simulink model "MPCHalo"  (R2019b)
settings: Solver=ode45  StartTime=0.0  StopTime=simTime  RelTol=1e-4
values from neighbouring files (symbols this model uses):
  a = zeros(2,1)    [initHaloMRMPC.m]
  b = zeros(2,1)    [initHaloMRMPC.m]
  c = zeros(2,1)    [initHaloMRMPC.m]
  delta = 0.1    [initHaloMRMPC.m]
  disturbance = 1    [initHaloMRMPC.m]
  Gsc = 1360.8    [initHaloMRMPC.m]
  k = 0.1    [initHaloMRMPC.m]
  L2 = 1.1556    [initHaloMRMPC.m]
  mu = 0.012149    [initHaloMRMPC.m]
  Omega = 1.8636    [initHaloMRMPC.m]
  Omega_z = Omega    (= 1.8636)    [initHaloMRMPC.m]
  phi = 0    [initHaloMRMPC.m]
  ref_select = 1    [initHaloMRMPC.m]
  Rotate_w = 0.1    [initHaloMRMPC.m]
  satValue = inf    [initHaloMRMPC.m]
  sped = 300000    [initHaloMRMPC.m]
  srp = 1    [initHaloMRMPC.m]
  Ts = delta    (= 0.1)    [initHaloMRMPC.m]
  u0 = [0;0;0]    [initHaloMRMPC.m]
  x0 = Seq + [ho1;diffho1]    [initHaloMRMPC.m]
  zeta = 0.9252    [initHaloMRMPC.m]
libraries: vrlib x3, mpclib x1, simulink x1
settings Model: Creator=mohd-  LastModifiedBy=mohd-

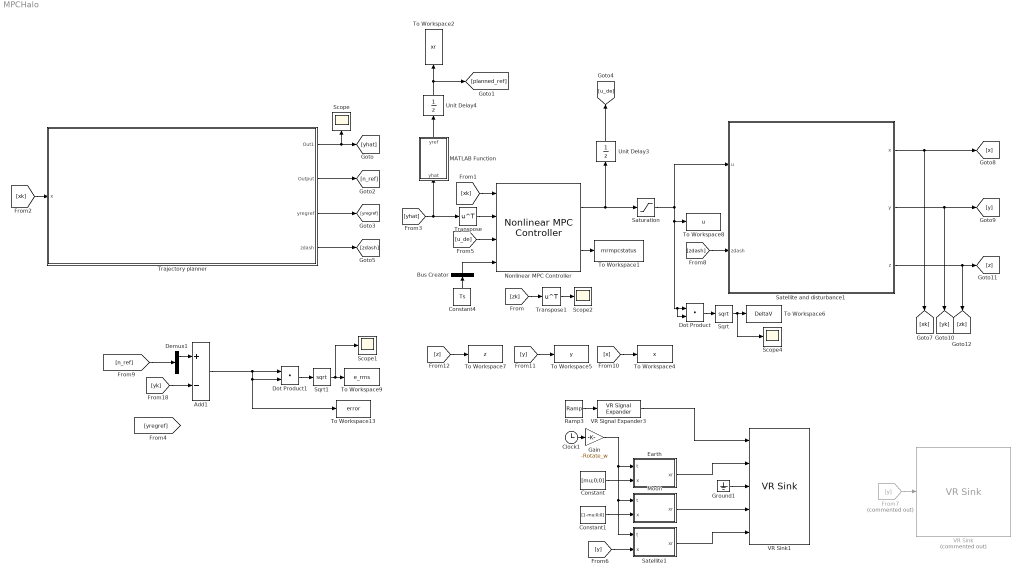
== system MPCHalo ==
  Add1 : Sum  Inputs=+-
  Bus Creator : BusCreator  Inputs=1  OutDataTypeStr=Bus: myBusObject  NonVirtualBus=on
      settings: InheritFromInputs=off
  Clock1 : Clock
  Constant : Constant  Value=[mu;0;0]
  Constant1 : Constant  Value=[1-mu;0;0]
  Constant4 : Constant  Value=Ts
  Demux1 : Demux  Outputs=[3 3]
  Dot Product : DotProduct  InputSameDT=on  OutDataTypeStr=Inherit: Inherit via internal rule
  Dot Product1 : DotProduct  InputSameDT=on  OutDataTypeStr=Inherit: Inherit via internal rule
  Earth : MATLAB Function  TreatAsAtomicUnit=on
  From7 : From  Commented=on  GotoTag=y
  Gain : Gain  Gain=-Rotate_w
  Ground1 : Ground
  MATLAB Function : MATLAB Function  TreatAsAtomicUnit=on
  Moon : MATLAB Function  TreatAsAtomicUnit=on
  Nonlinear MPC Controller : mpclib/Nonlinear MPC Controller  SCDEnableBlockLinearizationSpecification=on  nlmpcobj=nlobj  UseObjectTs=off  TsControl=delta  md_enabled=off  mvtarget_enabled=off  param_enabled=on  cost_enabled=off  mvseq_enabled=off  stateseq_enabled=off  ovseq_enabled=off  slack_enabled=off  status_enabled=on  ov_min=off  ov_max=off  mv_min=off  mv_max=off  mvrate_min=off  mvrate_max=off  state_min=off  state_max=off  ov_weight=off  mv_weight=off  mvrate_weight=off  ecr_weight=off  nlp_initialize=off
      settings: SourceProductName=Model Predictive Control Toolbox
  Ramp3 : simulink/Sources/Ramp  slope=0.4632  start=0  InitialOutput=0
  Satellite and disturbance1 : Subsystem
  Satellite1 : MATLAB Function  TreatAsAtomicUnit=on
  Saturation : Saturate  UpperLimit=satValue  LowerLimit=-satValue
  Scope{,1..2,4} (4 alike) : Scope
  Sqrt : Sqrt  SaturateOnIntegerOverflow=on
  Sqrt1 : Sqrt  SaturateOnIntegerOverflow=on
  To Workspace1 : ToWorkspace  VariableName=mrmpcstatus  SampleTime=10^-3
  To Workspace13 : ToWorkspace  VariableName=error  SampleTime=10^-3
  To Workspace2 : ToWorkspace  VariableName=xr  SampleTime=delta
  To Workspace4 : ToWorkspace  VariableName=x  SampleTime=10^-3
  To Workspace5 : ToWorkspace  VariableName=y  SampleTime=10^-3
  To Workspace6 : ToWorkspace  VariableName=DeltaV  SampleTime=10^-3
  To Workspace7 : ToWorkspace  VariableName=z  SampleTime=10^-3
  To Workspace8 : ToWorkspace  VariableName=u  SampleTime=10^-3
  To Workspace9 : ToWorkspace  VariableName=e_rms  SampleTime=delta
  Trajectory planner : Subsystem
  Transpose : Math  Operator=transpose  SignedPower=off  SaturateOnIntegerOverflow=on
  Transpose1 : Math  Operator=transpose  SignedPower=off  SaturateOnIntegerOverflow=on
  Unit Delay3 : UnitDelay  InitialCondition=u0  SampleTime=delta  HasFrameUpgradeWarning=on
  Unit Delay4 : UnitDelay  InitialCondition=x0  SampleTime=delta  HasFrameUpgradeWarning=on
  VR Signal Expander3 : vrlib/VR Signal Expander  outwidth=4  outidx=[4]
      settings: SourceProductName=Simulink
  VR Sink : vrlib/VR Sink  Commented=on  InstantiateOnLoad=on  SampleTime=-1  ViewEnable=on  RemoteChange=off  RemoteView=off  FieldsWritten=Satellite.translation.3.1.1.double  WorldFileName=satellite.wrl  WorldDescription=HaloMRMPC  AutoView=on  VideoDimensions=[]  AllowVariableSize=off  FigureProperties="{'Position', 'Name', 'Viewpoint', 'CameraBound', 'CameraDirection', 'CameraPosition', 'CameraUpVector', 'ZoomFactor', 'Antialiasing', 'Headlight', 'Lighting', 'NavPanel', 'Sound', 'StatusBar', 'Stereo3D', 'Stereo3DCameraOffset', 'Stereo3DHIT', 'ToolBar', 'Textures', 'Transparency', 'Triad', 'Wireframe', 'NavZones', 'NavMode', 'NavSpeed', 'CaptureFileFormat', 'CaptureFileName', 'Record2DCompressMethod', 'Record2DCompressQuality', 'Record2D', 'Record2DFileName', 'Record2DFPS'; [5.0000000000000000e+00   9.2000000000000000e+01   5.7600000000000000e+02   3.5000000000000000e+02], 'HaloMRMPC', 'View on Moon', 'on', [0.0000000000000000e+00   0.0000000000000000e+00  -1.0000000000000000e+00], [0.0000000000000000e+00   0.0000000000000000e+00   0.0000000000000000e+00], [0.0000000000000000e+00   1.0000000000000000e+00   0.0000000000000000e+00], [1.0000000000000000e+00], 'on', 'on', 'on', 'halfbar', 'on', 'on', 'off', [1.0000000149011612e-01], [0.0000000000000000e+00], 'on', 'on', 'on', 'none', 'off', 'off', 'fly', 'normal', 'tif', '%f_anim_%n.tif', 'auto', [7.5000000000000000e+01], 'off', '%f_anim_%n.avi', 'auto'}"
      settings: SourceProductName=Simulink
  VR Sink1 : vrlib/VR Sink  InstantiateOnLoad=on  SampleTime=-1  ViewEnable=on  RemoteChange=off  RemoteView=off  FieldsWritten=Earth.rotation.4.1.1.double#Earth.translation.3.1.1.double#Moon.rotation.4.1.1.double#Moon.translation.3.1.1.double#Satellite.translation.3.1.1.double  WorldFileName=satellite.wrl  WorldDescription=HaloMRMPC  AutoView=off  VideoDimensions=[]  AllowVariableSize=off
      settings: SourceProductName=Simulink
  wires:
  [z] -> To Workspace7/1
  [x] -> To Workspace4/1
  [y] -> To Workspace5/1
  Satellite and disturbance1/3(z) -> [z], [zk]
  Satellite and disturbance1/2(y) -> [yk], [y]
  Satellite and disturbance1/1(x) -> [xk], [x]
  Unit Delay3/1 -> [u_de]
  [u_de] -> Nonlinear MPC Controller/3
  [xk] -> Nonlinear MPC Controller/1
  Constant4/1 -> Bus Creator/1
  Bus Creator/1 -> Nonlinear MPC Controller/4
  Transpose/1 -> Nonlinear MPC Controller/2
  [zk] -> Transpose1/1
  Transpose1/1 -> Scope2/1
  [yk] -> Add1/2
  Dot Product/1 -> Sqrt/1
  Sqrt1/1 -> Scope1/1, To Workspace9/1
  Trajectory planner/1(Out1) -> [yhat], Scope/1
  [xk] -> Trajectory planner/1(x)
  MATLAB Function/1(yref) -> Unit Delay4/1
  Unit Delay4/1 -> [planned_ref], To Workspace2/1
  [yhat] -> MATLAB Function/1(yhat), Transpose/1
  Nonlinear MPC Controller/1 -> Unit Delay3/1, Saturation/1
  Saturation/1 -> Dot Product/1, Dot Product/2, To Workspace8/1, Satellite and disturbance1/1(u)
  Nonlinear MPC Controller/2 -> To Workspace1/1
  Sqrt/1 -> To Workspace6/1, Scope4/1
  Trajectory planner/2(Output) -> [n_ref]
  Dot Product1/1 -> Sqrt1/1
  Constant/1 -> Earth/2(x)
  Gain/1 -> Earth/1(t), Satellite1/1(t), Moon/1(t)
  Constant1/1 -> Moon/2(x)
  Clock1/1 -> Gain/1
  [y] -> Satellite1/2(x)
  Ramp3/1 -> VR Signal Expander3/1
  Satellite1/1(xr) -> VR Sink1/5
  Moon/1(xr) -> VR Sink1/4
  Earth/1(xr) -> VR Sink1/2
  VR Signal Expander3/1 -> VR Sink1/1
  Ground1/1 -> VR Sink1/3
  From7/1 -> VR Sink/1
  Trajectory planner/3("yregref ") -> [yregref]
  Trajectory planner/4("zdash ") -> [zdash]
  [zdash] -> Satellite and disturbance1/2("zdash ")
  [n_ref] -> Demux1/1
  Demux1/1 -> Add1/1
  Add1/1 -> To Workspace13/1, Dot Product1/2, Dot Product1/1

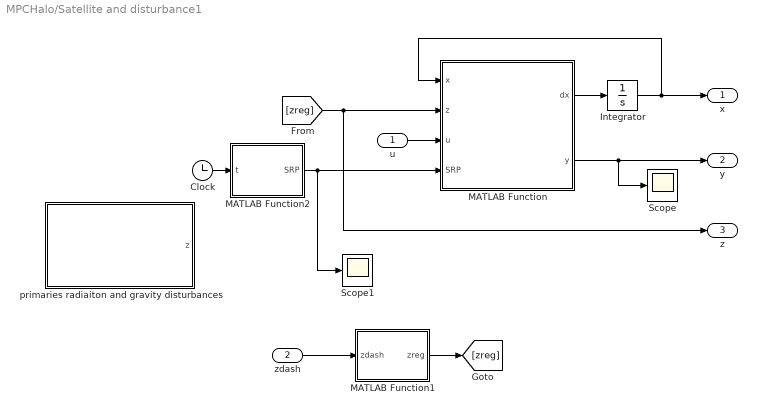
== system MPCHalo/Satellite and disturbance1 ==
  u : Inport
  "zdash " : Inport  Port=2
  Clock : Clock
  Integrator : Integrator  InitialCondition=x0
  MATLAB Function : MATLAB Function  TreatAsAtomicUnit=on
  MATLAB Function1 : MATLAB Function  TreatAsAtomicUnit=on
  MATLAB Function2 : MATLAB Function  TreatAsAtomicUnit=on
  Scope : Scope
  Scope1 : Scope
  primaries radiaiton and gravity disturbances : Subsystem
  x : Outport
  y : Outport  Port=2
  z : Outport  Port=3
  wires:
  Integrator/1 -> x/1, MATLAB Function/1(x)
  MATLAB Function/1(dx) -> Integrator/1
  MATLAB Function/2(y) -> Scope/1, y/1
  u/1 -> MATLAB Function/3(u)
  MATLAB Function1/1(zreg) -> [zreg]
  "zdash "/1 -> MATLAB Function1/1(zdash)
  [zreg] -> z/1, MATLAB Function/2(z)
  MATLAB Function2/1(SRP) -> Scope1/1, MATLAB Function/4(SRP)
  Clock/1 -> MATLAB Function2/1(t)

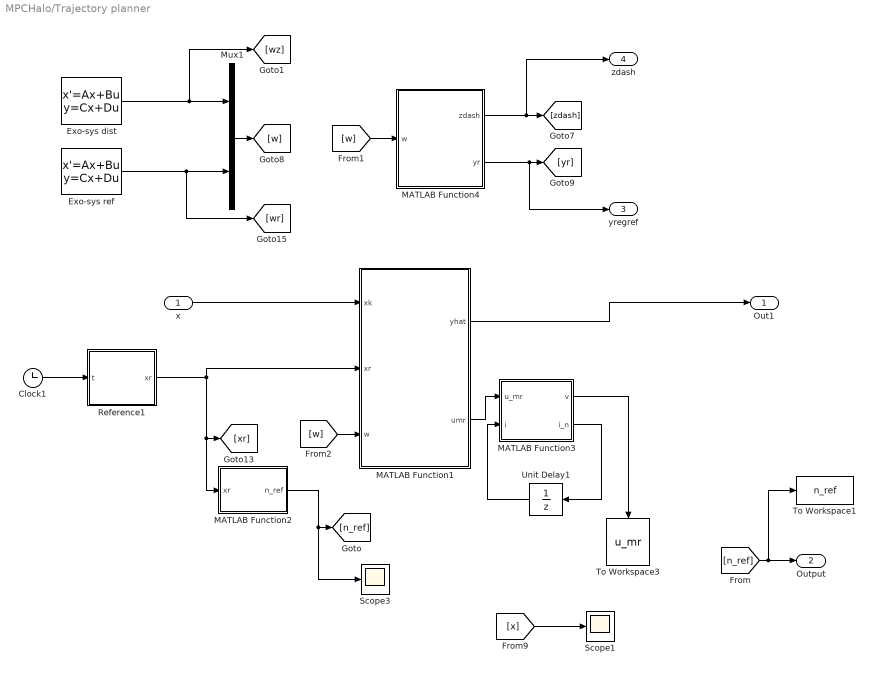
== system MPCHalo/Trajectory planner ==
  x : Inport
  Clock1 : Clock
  Exo-sys dist : StateSpace  A=[0 -1;1 0]  B=[0;0]  C=eye(2)  D=zeros(2,1)  InitialCondition=[1;0]
  "Exo-sys ref " : StateSpace  A=[0 -Omega;Omega 0]  B=[0;0]  C=eye(2)  D=zeros(2,1)  InitialCondition=[1;0]
  MATLAB Function1 : MATLAB Function  TreatAsAtomicUnit=on  SystemSampleTime=2*delta
  MATLAB Function2 : MATLAB Function  TreatAsAtomicUnit=on
  MATLAB Function3 : MATLAB Function  TreatAsAtomicUnit=on  SystemSampleTime=delta
  MATLAB Function4 : MATLAB Function  TreatAsAtomicUnit=on
  Mux1 : Mux  Inputs=2
  Reference1 : MATLAB Function  TreatAsAtomicUnit=on
  Scope1 : Scope
  Scope3 : Scope
  To Workspace1 : ToWorkspace  VariableName=n_ref  SampleTime=10^-3
  To Workspace3 : ToWorkspace  VariableName=u_mr  SampleTime=10^-3
  Unit Delay1 : UnitDelay  InitialCondition=1  SampleTime=delta  HasFrameUpgradeWarning=on
  Out1 : Outport
  Output : Outport  Port=2
  "yregref " : Outport  Port=3
  "zdash " : Outport  Port=4
  wires:
  MATLAB Function1/1(yhat) -> Out1/1
  Clock1/1 -> Reference1/1(t)
  x/1 -> MATLAB Function1/1(xk)
  MATLAB Function2/1(n_ref) -> Scope3/1, [n_ref]
  Unit Delay1/1 -> MATLAB Function3/2(i)
  MATLAB Function1/2(umr) -> MATLAB Function3/1(u_mr)
  [x] -> Scope1/1
  Reference1/1(xr) -> MATLAB Function2/1(xr), [xr], MATLAB Function1/2(xr)
  MATLAB Function3/2(i_n) -> Unit Delay1/1
  MATLAB Function3/1(v) -> To Workspace3/1
  [n_ref] -> To Workspace1/1, Output/1
  MATLAB Function4/1(zdash) -> "zdash "/1, [zdash]
  MATLAB Function4/2(yr) -> "yregref "/1, [yr]
  Mux1/1 -> [w]
  Exo-sys dist/1 -> [wz], Mux1/1
  [w] -> MATLAB Function4/1(w)
  "Exo-sys ref "/1 -> [wr], Mux1/2
  [w] -> MATLAB Function1/3(w)

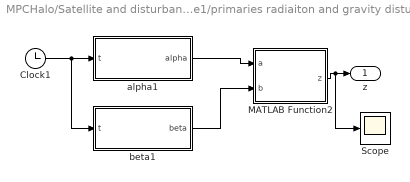
== system MPCHalo/Satellite and disturbance1/primaries radiaiton and gravity disturbances ==
  Clock1 : Clock
  MATLAB Function2 : MATLAB Function  TreatAsAtomicUnit=on
  Scope : Scope
  alpha1 : MATLAB Function  TreatAsAtomicUnit=on
  beta1 : MATLAB Function  TreatAsAtomicUnit=on
  z : Outport
  wires:
  Clock1/1 -> beta1/1(t), alpha1/1(t)
  beta1/1(beta) -> MATLAB Function2/2(b)
  alpha1/1(alpha) -> MATLAB Function2/1(a)
  MATLAB Function2/1(z) -> Scope/1, z/1

== matlab function MPCHalo/Trajectory planner/MATLAB Function2 ==
  data: xr input; n_ref output
function n_ref = fcn(xr)

n_ref = xr(:,1);

== matlab function MPCHalo/MATLAB Function ==
  data: yhat input; yref output
function yref = fcn(yhat)

yref = yhat(:,1);

== matlab function MPCHalo/Earth ==
  data: t input; xr output; x input
function xr = Rotate(t,x)
%#codegen

th = t;

R = [cos(th) sin(th) 0;
     -sin(th) cos(th) 0;
     0 0 1];
xr = R*x;

== matlab function MPCHalo/Trajectory planner/MATLAB Function1 ==
  data: yhat output; xk input; umr output; xr input; mu parameter; delta parameter; c parameter; w input; k parameter; e parameter; a parameter; b parameter; Omega parameter; disturbance parameter; L2 parameter
function [yhat, umr] = mrcontrol(xk,xr, mu,delta,c, w,k, e, a, b, Omega, disturbance, L2)

Tz = [b(1)*e 0;0 0;0 -b(1)*e;mu*(1-mu)*a(1)*e 0];
Tr = [k*(1-c(1)+Omega^2)/(2*Omega) 0;0 -k;-k 0];
S2 = [0 -Omega;Omega 0];
Seq = [L2;0;0];
if disturbance == 1
    wz = w(1:2);
else
    wz = zeros(2,1);
end
wr = w(3:4);
pi = [-Tr*wr + Seq;-Tr*S2*wr];

% ref1 = xr(:,1);
% ref2 = xr(:,2);
ref1 = pi;
ref2 = ref1;

u = zeros(3,2);
yhat = zeros(6,4); % 3 outputs for 4 small time intervals (2*delta)
x_t = xk;

delta_b = delta;
%% First step 

Ad = [ 1, 0, 0, delta_b, 0, 0; ...
      0, 1, 0, 0, delta_b,  0; ...
      0, 0, 1, 0, 0, delta_b; ...
      0, 0, 0, 1, 0,  0; ...
      0, 0, 0, 0, 1, 0; ...
      0, 0, 0, 0, 0, 1];
Am = Ad^2;
  
Bd = [delta_b^2/2 0 0;0 delta_b^2/2 0;0 0 delta_b^2/2; ...
       delta_b 0 0;0 delta_b 0; 0 0 delta_b];

Bm = [Ad*Bd Bd]; 
Cm = [eye(3) zeros(3)];

u1 = pinv(Bm)*(ref1-Am*xk);  
u11 = u1(1); 
u21 = u1(2);
u31 = u1(3);
u12 = u1(4);
u22 = u1(5);
u32 = u1(6);

u_1 = [u11 u12;u21 u22;u31 u32];

%% Second step 
xk1 = Am*xk + Bm*u1;  
u2 = pinv(Bm)*(ref2-Am*xk1); 

u11 = u2(1); 
u21 = u2(2);
u31 = u2(3);
u12 = u2(4);
u22 = u2(5);
u32 = u2(6);

u_2 = [u11 u12;u21 u22;u31 u32];

%% States planning step

x_1 = pi(1);
x_2 = pi(2);
x_3 = pi(3);
xd_1 = pi(4);
xd_2 = pi(5);


f2 = [x_1 + 2*xd_2 - (mu*(mu + x_1 - 1))/((mu + x_1 - 1)^2 + x_2^2 + x_3^2)^(3/2) + ((mu + x_1)*(mu - 1))/((mu + x_1)^2 + x_2^2 + x_3^2)^(3/2);
    x_2 - 2*xd_1 - (mu*x_2)/((mu + x_1 - 1)^2 + x_2^2 + x_3^2)^(3/2) + (x_2*(mu - 1))/((mu + x_1)^2 + x_2^2 + x_3^2)^(3/2);
    (x_3*(mu - 1))/((mu + x_1)^2 + x_2^2 + x_3^2)^(3/2) - (mu*x_3)/((mu + x_1 - 1)^2 + x_2^2 + x_3^2)^(3/2)];

P44 = -2*((x_1+mu)^2+x_2^2+x_3^2)/((x_1+mu)^2+x_2^2+x_3^2)^(5/2) - 2*((x_1-1+mu)^2+x_2^2+x_3^2)/((x_1-1+mu)^2+x_2^2+x_3^2)^(5/2);
P54 = 3*(x_2*(x_1+mu))/((x_1+mu)^2+x_2^2+x_3^2)^(5/2) - 3*(x_2*(x_1-1+mu))/((x_1-1+mu)^2+x_2^2+x_3^2)^(5/2);
P64 = 3*(x_3*(x_1+mu))/((x_1+mu)^2+x_2^2+x_3^2)^(5/2) - 3*x_3*((x_1-1+mu))/((x_1-1+mu)^2+x_2^2+x_3^2)^(5/2);

P2 = [ 2*x_1 + 2*xd_2, x_1,  x_2, P44;
    2*x_2 - 2*xd_1, x_2, -x_1, P54;
    0,   0,    0, P64];

gamma_d = - f2 - P2*Tz*wz - Tr*S2^2*wr;

G  = [zeros(3,3);eye(3)];

%% step one

x_1 = xk(1);
x_2 = xk(2);
x_3 = xk(3);
xd_1 = xk(4);
xd_2 = xk(5);


f2 = [x_1 + 2*xd_2 - (mu*(mu + x_1 - 1))/((mu + x_1 - 1)^2 + x_2^2 + x_3^2)^(3/2) + ((mu + x_1)*(mu - 1))/((mu + x_1)^2 + x_2^2 + x_3^2)^(3/2);
    x_2 - 2*xd_1 - (mu*x_2)/((mu + x_1 - 1)^2 + x_2^2 + x_3^2)^(3/2) + (x_2*(mu - 1))/((mu + x_1)^2 + x_2^2 + x_3^2)^(3/2);
    (x_3*(mu - 1))/((mu + x_1)^2 + x_2^2 + x_3^2)^(3/2) - (mu*x_3)/((mu + x_1 - 1)^2 + x_2^2 + x_3^2)^(3/2)];

P44 = -2*((x_1+mu)^2+x_2^2+x_3^2)/((x_1+mu)^2+x_2^2+x_3^2)^(5/2) - 2*((x_1-1+mu)^2+x_2^2+x_3^2)/((x_1-1+mu)^2+x_2^2+x_3^2)^(5/2);
P54 = 3*(x_2*(x_1+mu))/((x_1+mu)^2+x_2^2+x_3^2)^(5/2) - 3*(x_2*(x_1-1+mu))/((x_1-1+mu)^2+x_2^2+x_3^2)^(5/2);
P64 = 3*(x_3*(x_1+mu))/((x_1+mu)^2+x_2^2+x_3^2)^(5/2) - 3*x_3*((x_1-1+mu))/((x_1-1+mu)^2+x_2^2+x_3^2)^(5/2);

P2 = [ 2*x_1 + 2*xd_2, x_1,  x_2, P44;
    2*x_2 - 2*xd_1, x_2, -x_1, P54;
    0,   0,    0, P64];


% Cd = Cm;
% x = x_t;

F = [xk(4:6);f2];
P = [zeros(3,4);P2];
x1 = xk + delta_b*(F + P*Tz*wz + G*(gamma_d + u_1(:,1)));
yhat(:,1) = x1;


%% step two
x_1 = x1(1);
x_2 = x1(2);
x_3 = x1(3);
xd_1 = x1(4);
xd_2 = x1(5);


f2 = [x_1 + 2*xd_2 - (mu*(mu + x_1 - 1))/((mu + x_1 - 1)^2 + x_2^2 + x_3^2)^(3/2) + ((mu + x_1)*(mu - 1))/((mu + x_1)^2 + x_2^2 + x_3^2)^(3/2);
    x_2 - 2*xd_1 - (mu*x_2)/((mu + x_1 - 1)^2 + x_2^2 + x_3^2)^(3/2) + (x_2*(mu - 1))/((mu + x_1)^2 + x_2^2 + x_3^2)^(3/2);
    (x_3*(mu - 1))/((mu + x_1)^2 + x_2^2 + x_3^2)^(3/2) - (mu*x_3)/((mu + x_1 - 1)^2 + x_2^2 + x_3^2)^(3/2)];

P44 = -2*((x_1+mu)^2+x_2^2+x_3^2)/((x_1+mu)^2+x_2^2+x_3^2)^(5/2) - 2*((x_1-1+mu)^2+x_2^2+x_3^2)/((x_1-1+mu)^2+x_2^2+x_3^2)^(5/2);
P54 = 3*(x_2*(x_1+mu))/((x_1+mu)^2+x_2^2+x_3^2)^(5/2) - 3*(x_2*(x_1-1+mu))/((x_1-1+mu)^2+x_2^2+x_3^2)^(5/2);
P64 = 3*(x_3*(x_1+mu))/((x_1+mu)^2+x_2^2+x_3^2)^(5/2) - 3*x_3*((x_1-1+mu))/((x_1-1+mu)^2+x_2^2+x_3^2)^(5/2);

P2 = [ 2*x_1 + 2*xd_2, x_1,  x_2, P44;
    2*x_2 - 2*xd_1, x_2, -x_1, P54;
    0,   0,    0, P64];


% Cd = Cm;
% x = x_t;

F = [x1(4:6);f2];
P = [zeros(3,4);P2];

x2 = x1 + delta_b*(F + P*Tz*wz + G*(gamma_d + u_1(:,2)));
yhat(:,2) = x2;


%% third step 
x_1 = x2(1);
x_2 = x2(2);
x_3 = x2(3);
xd_1 = x2(4);
xd_2 = x2(5);


f2 = [x_1 + 2*xd_2 - (mu*(mu + x_1 - 1))/((mu + x_1 - 1)^2 + x_2^2 + x_3^2)^(3/2) + ((mu + x_1)*(mu - 1))/((mu + x_1)^2 + x_2^2 + x_3^2)^(3/2);
    x_2 - 2*xd_1 - (mu*x_2)/((mu + x_1 - 1)^2 + x_2^2 + x_3^2)^(3/2) + (x_2*(mu - 1))/((mu + x_1)^2 + x_2^2 + x_3^2)^(3/2);
    (x_3*(mu - 1))/((mu + x_1)^2 + x_2^2 + x_3^2)^(3/2) - (mu*x_3)/((mu + x_1 - 1)^2 + x_2^2 + x_3^2)^(3/2)];

P44 = -2*((x_1+mu)^2+x_2^2+x_3^2)/((x_1+mu)^2+x_2^2+x_3^2)^(5/2) - 2*((x_1-1+mu)^2+x_2^2+x_3^2)/((x_1-1+mu)^2+x_2^2+x_3^2)^(5/2);
P54 = 3*(x_2*(x_1+mu))/((x_1+mu)^2+x_2^2+x_3^2)^(5/2) - 3*(x_2*(x_1-1+mu))/((x_1-1+mu)^2+x_2^2+x_3^2)^(5/2);
P64 = 3*(x_3*(x_1+mu))/((x_1+mu)^2+x_2^2+x_3^2)^(5/2) - 3*x_3*((x_1-1+mu))/((x_1-1+mu)^2+x_2^2+x_3^2)^(5/2);

P2 = [ 2*x_1 + 2*xd_2, x_1,  x_2, P44;
    2*x_2 - 2*xd_1, x_2, -x_1, P54;
    0,   0,    0, P64];


% Cd = Cm;
% x = x_t;

F = [x2(4:6);f2];
P = [zeros(3,4);P2];

x3 = x2 + delta_b*(F + P*Tz*wz + G*(gamma_d + u_2(:,1)));
yhat(:,3) = x3;


%% fourth step
x_1 = x3(1);
x_2 = x3(2);
x_3 = x3(3);
xd_1 = x3(4);
xd_2 = x3(5);


f2 = [x_1 + 2*xd_2 - (mu*(mu + x_1 - 1))/((mu + x_1 - 1)^2 + x_2^2 + x_3^2)^(3/2) + ((mu + x_1)*(mu - 1))/((mu + x_1)^2 + x_2^2 + x_3^2)^(3/2);
    x_2 - 2*xd_1 - (mu*x_2)/((mu + x_1 - 1)^2 + x_2^2 + x_3^2)^(3/2) + (x_2*(mu - 1))/((mu + x_1)^2 + x_2^2 + x_3^2)^(3/2);
    (x_3*(mu - 1))/((mu + x_1)^2 + x_2^2 + x_3^2)^(3/2) - (mu*x_3)/((mu + x_1 - 1)^2 + x_2^2 + x_3^2)^(3/2)];

P44 = -2*((x_1+mu)^2+x_2^2+x_3^2)/((x_1+mu)^2+x_2^2+x_3^2)^(5/2) - 2*((x_1-1+mu)^2+x_2^2+x_3^2)/((x_1-1+mu)^2+x_2^2+x_3^2)^(5/2);
P54 = 3*(x_2*(x_1+mu))/((x_1+mu)^2+x_2^2+x_3^2)^(5/2) - 3*(x_2*(x_1-1+mu))/((x_1-1+mu)^2+x_2^2+x_3^2)^(5/2);
P64 = 3*(x_3*(x_1+mu))/((x_1+mu)^2+x_2^2+x_3^2)^(5/2) - 3*x_3*((x_1-1+mu))/((x_1-1+mu)^2+x_2^2+x_3^2)^(5/2);

P2 = [ 2*x_1 + 2*xd_2, x_1,  x_2, P44;
    2*x_2 - 2*xd_1, x_2, -x_1, P54;
    0,   0,    0, P64];


% Cd = Cm;
% x = x_t;

F = [x3(4:6);f2];
P = [zeros(3,4);P2];

x4 = x3 + delta_b*(F + P*Tz*wz + G*(gamma_d + u_2(:,2)));
yhat(:,4) = x4;


umr = u_1;

== matlab function MPCHalo/Satellite1 ==
  data: t input; xr output; x input
function xr = Rotate(t,x)
%#codegen

th = t;

R = [cos(th) sin(th) 0;
     -sin(th) cos(th) 0;
     0 0 1];
 
xr = R*x;

== matlab function MPCHalo/Trajectory planner/MATLAB Function4 ==
  data: zdash output; w input; yr output; c parameter; Omega parameter; k parameter; a parameter; b parameter; mu parameter; e parameter; L2 parameter
function [zdash,yr] = fcn(w, c, Omega, k, a, b, mu, e, L2)

Seq = [L2;0;0];

T1 = [b(1)*e 0;0 0;0 -b(1)*e;mu*(1-mu)*a(1)*e 0];
Q1 = [k*(1-c(1)+Omega^2)/(2*Omega) 0;0 -k;-k 0];

zdash = T1*w(1:2);
yr = Q1*w(3:4) + Seq;

== matlab function MPCHalo/Moon ==
  data: t input; xr output; x input
function xr = Rotate(t,x)
%#codegen

th = t;

R = [cos(th) sin(th) 0;
     -sin(th) cos(th) 0;
     0 0 1];

xr = R*x;

== matlab function MPCHalo/Satellite and disturbance1/MATLAB Function1 ==
  data: zdash input; zreg output; disturbance parameter
function zreg = fcn(zdash, disturbance)

if disturbance == 1 
    zreg = zdash;
else
    zreg = zeros(4,1);
end

== matlab function MPCHalo/Trajectory planner/MATLAB Function3 ==
  data: u_mr input; v output; i input size=1; i_n output size=1
function [v,i_n] = fcn(u_mr, i)
if i <2
    i_n = i+1; 
else
    i_n = 1;
end

v = u_mr(:, i);

== matlab function MPCHalo/Trajectory planner/Reference1 ==
  data: t input; xr output; c parameter; Omega parameter; Omega_z parameter; L2 parameter; k parameter; delta parameter; ref_select parameter; e parameter
function xr = refer(t,c,Omega,Omega_z,L2,k,delta,ref_select,e)
%#codegen

% delta = 2*delta_b;
Seq = [L2;0;0;0;0;0];


ho1 = [(-k*(1-c(1)+Omega^2)/(2*Omega))*cos(Omega*t);
       k*sin(Omega*t);
       k*cos(Omega_z*t)];
   
diffho1 = [(k*(1-c(1)+Omega^2)/2)*sin(Omega*t);
           Omega*k*cos(Omega*t);
           -Omega_z*k*sin(Omega_z*t)];
      
% Halo orbit reference type 1       
% xr = Seq;
% if (ref_select == 1) 
    xr1 = Seq + [ho1;diffho1];

    ho11 = [(-k*(1-c(1)+Omega^2)/(2*Omega))*cos(Omega*(t+delta));
           k*sin(Omega*(t+delta));
           k*cos(Omega_z*(t+delta))];

    diffho11 = [(k*(1-c(1)+Omega^2)/2)*sin(Omega*(t+delta));
               Omega*k*cos(Omega*(t+delta));
               -Omega_z*k*sin(Omega_z*(t+delta))];

    xr2 = Seq + [ho11;diffho11];

    xr = [xr1 xr2];
%     else
%     xr = [L2 L2;0 0;0 0;0 0;0 0;0 0];
%end


% xr = xr1(1:6);

== matlab function MPCHalo/Satellite and disturbance1/MATLAB Function ==
  data: x input; z input; dx output; u input; y output; mu parameter; SRP input
function [dx, y] = Satellite(x,z, u, mu, SRP)

x1 = x(1:3);
x2 = x(4:6);

M = [-1 0 0;
    0 -1 0;
    0 0 0];

N = [0 -1 0;
    1 0 0;
    0 0 0];

d1r = [-mu - z(4)/(1-mu);0;0];
d2r = [1-mu + z(4)/mu;0;0];

ed1 = x1 - d1r;
absed1 = sqrt(ed1(1)^2+ed1(2)^2+ed1(3)^2);
ed2 = x1 - d2r;
absed2 = sqrt(ed2(1)^2+ed2(2)^2+ed2(3)^2);

f1 = x2;
f2 = -M*x1 - 2*N*x2 - (2*M*x1 + 2*N*x2)*z(1) ...
           - M*x1*z(2) - N*x1*z(3) - ed1*(1 - mu)/absed1^3 ...
           - ed2*mu/absed2^3;
F = [f1; f2 + SRP];
G = [zeros(3); eye(3)];


dx = F + G*u;
y  = x1;

%% simplified model
% x_1 = x1(1);
% x_2 = x1(2);
% x_3 = x1(3);
% xd_1 = x2(1);
% xd_2 = x2(2);
% xd_3 = x2(3);
% % 
% f2 = [x_1 + 2*xd_2 - (mu*(mu + x_1 - 1))/((mu + x_1 - 1)^2 + x_2^2 + x_3^2)^(3/2) + ((mu + x_1)*(mu - 1))/((mu + x_1)^2 + x_2^2 + x_3^2)^(3/2);
%     x_2 - 2*xd_1 - (mu*x_2)/((mu + x_1 - 1)^2 + x_2^2 + x_3^2)^(3/2) + (x_2*(mu - 1))/((mu + x_1)^2 + x_2^2 + x_3^2)^(3/2);
%     (x_3*(mu - 1))/((mu + x_1)^2 + x_2^2 + x_3^2)^(3/2) - (mu*x_3)/((mu + x_1 - 1)^2 + x_2^2 + x_3^2)^(3/2)];
% 
% F = [x2; f2];
% 
% P44 = -2*((x_1+mu)^2+x_2^2+x_3^2)/((x_1+mu)^2+x_2^2+x_3^2)^(5/2) - 2*((x_1-1+mu)^2+x_2^2+x_3^2)/((x_1-1+mu)^2+x_2^2+x_3^2)^(5/2);
% P54 = 3*(x_2*(x_1+mu))/((x_1+mu)^2+x_2^2+x_3^2)^(5/2) - 3*(x_2*(x_1-1+mu))/((x_1-1+mu)^2+x_2^2+x_3^2)^(5/2);
% P64 = 3*(x_3*(x_1+mu))/((x_1+mu)^2+x_2^2+x_3^2)^(5/2) - 3*x_3*((x_1-1+mu))/((x_1-1+mu)^2+x_2^2+x_3^2)^(5/2);
% 
% P = [ 2*x_1 + 2*xd_2, x_1,  x_2, P44;
%     2*x_2 - 2*xd_1, x_2, -x_1, P54;
%     0,   0,    0, P64];
% 
% f = F + [zeros(3,4);P]*z;
% G = [zeros(3); eye(3)];
% dx = f + G*u;
% y = x1;

== matlab function MPCHalo/Satellite and disturbance1/primaries radiaiton and gravity disturbances/MATLAB Function2 ==
  data: a input; z output; b input; mu parameter; disturbance parameter
function z = z(a,b,mu, disturbance)
%#codegen
if disturbance == 1
    z = [b;mu*(1-mu)*a];
else
    z = zeros(4,1);
end

== matlab function MPCHalo/Satellite and disturbance1/primaries radiaiton and gravity disturbances/alpha1 ==
  data: t input; alpha output; a parameter; phi parameter; e parameter
function alpha = a(t,a,phi,e)
%#codegen

a1 = a(1)*e*cos(t+phi);
alpha = a1;

== matlab function MPCHalo/Satellite and disturbance1/primaries radiaiton and gravity disturbances/beta1 ==
  data: t input; beta output; b parameter; phi parameter; e parameter
function beta = b(t,b,phi,e)
%#codegen
b1 = b(1)*e*cos(t+phi);
bd = -b(1)*e*sin(t+phi);
beta = [b1;0;bd];

== matlab function MPCHalo/Satellite and disturbance1/MATLAB Function2 ==
  data: SRP output; srp parameter; Gsc parameter; sped parameter; zeta parameter; t input
function SRP = fcn(srp, Gsc, sped, zeta,t)

if srp == 1
    SRP = [(Gsc/sped)*(cos(zeta*t))^2;(Gsc/sped)*(sin(zeta*t))^2;0];
else
    SRP = [0;0;0];
end
